simulink model "Exercise_5"  (R2022a)
settings: Solver=FixedStepAuto  StartTime=0.0  StopTime=10.0  FixedStep=0.0001  RelTol=1e-3
settings Model: Creator=Shocky  LastModifiedBy=Shocky

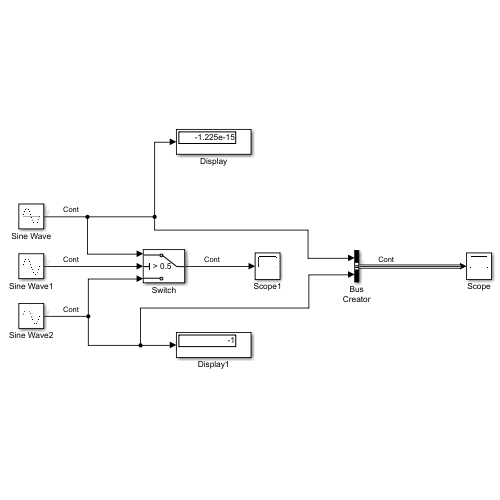
[thumbnail: Simulink's stored preview of the top-level diagram]
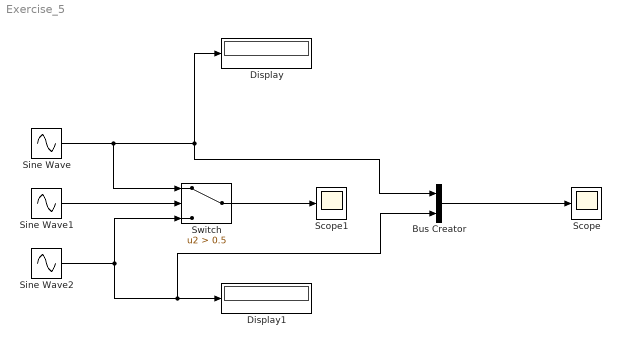
== system Exercise_5 ==
  Bus Creator : BusCreator  Inputs=2
  Display : Display
  Display1 : Display
  Scope : Scope
  Scope1 : Scope
  Sine Wave : Sin  Frequency=pi  SampleTime=0  VectorParams1D=off
  Sine Wave1 : Sin  Frequency=pi  SampleTime=0  VectorParams1D=off
  Sine Wave2 : Sin  Frequency=pi  Phase=-0.5*pi  SampleTime=0  VectorParams1D=off
  Switch : Switch  Criteria=u2 > Threshold  Threshold=0.5  SaturateOnIntegerOverflow=off  InputSameDT=off
  wires:
  Sine Wave/1 -> Bus Creator/1, Display/1, Switch/1
  Sine Wave1/1 -> Switch/2
  Sine Wave2/1 -> Switch/3, Bus Creator/2, Display1/1
  Switch/1 -> Scope1/1
  Bus Creator/1 -> Scope/1
